simulink model "test_euler_to_rw"  (R2022b)
settings: Solver=VariableStepAuto  StartTime=0.0  StopTime=10.0  RelTol=1e-3
settings Model: Creator=Jon  LastModifiedBy=Jon

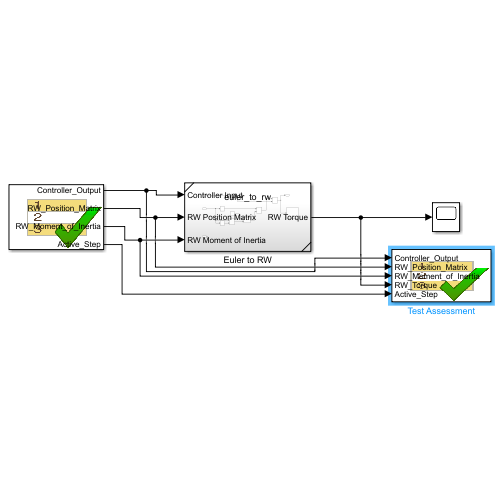
[thumbnail: Simulink's stored preview of the top-level diagram]
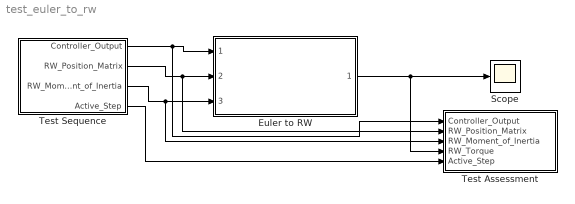
== system test_euler_to_rw ==
  Euler to RW : Subsystem  ReferencedSubsystem=euler_to_rw
  Scope : Scope
  Test Assessment : Test Sequence  TreatAsAtomicUnit=on
  Test Sequence : Test Sequence  TreatAsAtomicUnit=on
  wires:
  Euler to RW/1 -> Scope/1, Test Assessment/4(RW_Torque)
  Test Sequence/1(Controller_Output) -> Test Assessment/1(Controller_Output), Euler to RW/1
  Test Sequence/2(RW_Position_Matrix) -> Test Assessment/2(RW_Position_Matrix), Euler to RW/2
  Test Sequence/3(RW_Moment_of_Inertia) -> Test Assessment/3(RW_Moment_of_Inertia), Euler to RW/3
  Test Sequence/4(Active_Step) -> Test Assessment/5(Active_Step)

== stateflow chart test_euler_to_rw/Test Assessment ==
  state Assess_Any
    A = RW_Position_Matrix;
    verify(all(RW_Torque == transpose(A)*inv(A*transpose(A))*Controller_Output));
  (default) -> Assess_Any
  data: Controller_Output input; RW_Position_Matrix input; RW_Moment_of_Inertia input; RW_Torque input; Active_Step input; A local

== stateflow chart test_euler_to_rw/Test Sequence ==
  state Parallel_to_RW
    Controller_Output = [1; 1; -1];
    RW_Position_Matrix = 1/sqrt(3)*[[1;1;-1],[1;-1;-1],[-1;-1;-1],[-1;1;-1]];
    RW_Moment_of_Inertia = 1;
    settings: description=Test output when desired torque is parallel to the axis of a RW
  state Fully_Down
    Controller_Output = [0; 0; -1];
    settings: description=Test output when desired torque is straight down
  (default) -> Parallel_to_RW
  Parallel_to_RW -> Fully_Down : [
      | after(5, 'sec')
      | ]
  data: Controller_Output output; RW_Position_Matrix output; RW_Moment_of_Inertia output; Active_Step output string
